simulink model "dc_motor_model_h_bridge_feedforward"  (Simulink 7.8)
settings: Solver=ode15s  StartTime=0.0  StopTime=10.0  MaxStep=1  RelTol=1e-3
values from neighbouring files (symbols this model uses):
  J = 8.85*10^(-7)    (= 8.85e-07)    [dc_motor_basic_blocks_feedforward.m]    (also in dc_motor_basic_blocks_feedforward_test.m; dc_motor_h_bridge_feedforward.m)
  T_load = 0.1    [dc_motor_basic_blocks_feedforward.m]    (also in dc_motor_basic_blocks_feedforward_test.m; dc_motor_h_bridge_feedforward.m)
  U_d = (R*mu/k_tau + k_emf) * w_d + R/k_tau * T_load + R*J/k_tau*w_d_dot    (= 34.1839823009)    [dc_motor_basic_blocks_feedforward.m]    (also in dc_motor_basic_blocks_feedforward_test.m; dc_motor_h_bridge_feedforward.m)
libraries: fl_lib x6, nesl_utility x6, elec_lib x3
settings Model: Creator=krzysztof  LastModifiedBy=krzysztof

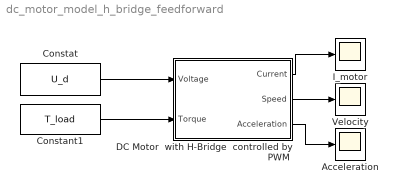
== system dc_motor_model_h_bridge_feedforward ==
  Acceleration : Scope
      settings: SaveName=Acceleration
  Constant1 : Constant  Value=T_load
  Constat : Constant  Value=U_d
  DC Motor  with H-Bridge  controlled by PWM : Subsystem
  I_motor : Scope
      settings: SaveName=i_motor
  Velocity : Scope
      settings: SaveName=w
  wires:
  DC Motor  with H-Bridge  controlled by PWM/1(Current) -> I_motor/1
  DC Motor  with H-Bridge  controlled by PWM/2(Speed) -> Velocity/1
  DC Motor  with H-Bridge  controlled by PWM/3(Acceleration) -> Acceleration/1
  Constat/1 -> DC Motor  with H-Bridge  controlled by PWM/1(Voltage)
  Constant1/1 -> DC Motor  with H-Bridge  controlled by PWM/2(Torque)

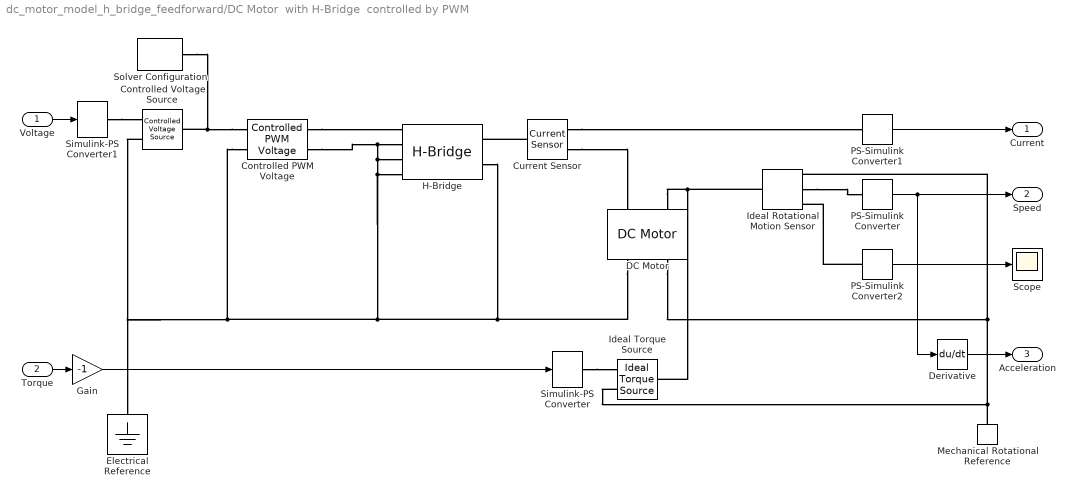
== system dc_motor_model_h_bridge_feedforward/DC Motor  with H-Bridge  controlled by PWM ==
  Voltage : Inport
  Torque : Inport  Port=2
  Controlled PWM Voltage : elec_lib/Actuators & Drivers/Drivers/Controlled PWM Voltage  F=f_PWM Hz  Vmin=Vmin V  Vmax=Vmax V  Vm=Vout V  pwm_or_av=2  current_Log=off  voltage_Log=off  power_Log=off  LocalVarNames=|current|voltage|power  LocalVarDescs=|Load current (A)|Load voltage (V)|Load power (W)  LocalVarLogging=[0 0 0]
  Controlled Voltage Source : fl_lib/Electrical/Electrical Sources/Controlled Voltage Source  i_Log=off  v_Log=off  LocalVarNames=|i|v  LocalVarDescs=|i|v  LocalVarLogging=[0 0]
  Current Sensor : fl_lib/Electrical/Electrical Sensors/Current Sensor  i1_Log=off  v1_Log=off  LocalVarNames=|i1|v1  LocalVarDescs=|i1|v1  LocalVarLogging=[0 0]
  DC Motor : elec_lib/Actuators & Drivers/Rotational Actuators/DC Motor  parameterization=2  Ra=3.9 Ohm  La=L H  emf_or_torque=1  Kv=7.2e-5 V/rpm  Ki=6.876e-4 N*m/A  T_stall=t_stall N*m  w_max=v_nl rad/s  w_rated=4070 rpm  P_rated=10 W  V_rated=Un V  J=J kg*m^2  lam_param=1  lam=mu N*m/(rad/s)  i_noload=I_nl A  V_i_noload=Un V  speed0=v0 rad/s  current_Log=off  voltage_Log=off  power_Log=off  i2r_Log=off  torque_Log=off  speed_Log=off  LocalVarNames=|current|voltage|power|i2r|torque|speed  LocalVarDescs=|Current (A)|Voltage (V)|Power (W)|Electrical losses (W)|Torque (Nm)|Angular speed (rad/s)  LocalVarLogging=[0 0 0 0 0 0]
  Derivative : Derivative
  Electrical Reference : fl_lib/Electrical/Electrical Elements/Electrical Reference  i_Log=off  LocalVarNames=|i  LocalVarDescs=|i  LocalVarLogging=0
  Gain : Gain  Gain=-1
  H-Bridge : elec_lib/Actuators & Drivers/Drivers/H-Bridge  Venable=in_en_tresh V  Vmax=in_pwm V  Vreverse=in_rev_tresh V  Vbrake=in_br_tresh V  Vm=h_Vout V  pwm_or_av=2  discontinuous=0  freewheeling_mode=1  freewheeling_mode_disc=1  Ron=h_res Ohm  Don=h_diode Ohm  Rload=10 Ohm  Lload=1e-5 H  F=10 kHz  current_Log=off  voltage_Log=off  power_Log=off  LocalVarNames=|current|voltage|power  LocalVarDescs=|Load current (A)|Load voltage (V)|Load power (W)  LocalVarLogging=[0 0 0]
  Ideal Rotational Motion Sensor : fl_lib/Mechanical/Mechanical Sensors/Ideal Rotational Motion Sensor  offset=0 rad  w_Log=off  t_Log=off  phi_Log=off  LocalVarNames=|w|t|phi  LocalVarDescs=|w|t|phi  LocalVarLogging=[0 0 0]
  Ideal Torque Source : fl_lib/Mechanical/Mechanical Sources/Ideal Torque Source  w_Log=off  t_Log=off  LocalVarNames=|w|t  LocalVarDescs=|w|t  LocalVarLogging=[0 0]
  Mechanical Rotational Reference : fl_lib/Mechanical/Rotational Elements/Mechanical Rotational Reference  t_Log=off  LocalVarNames=|t  LocalVarDescs=|t  LocalVarLogging=0
  PS-Simulink Converter : nesl_utility/PS-Simulink Converter  PhysicalDomain=network_engine_domain  LeftPortType=input  RightPortType=output  SubClassName=ps_output  Unit=rad/s  AffineConversion=off
  PS-Simulink Converter1 : nesl_utility/PS-Simulink Converter  PhysicalDomain=network_engine_domain  LeftPortType=input  RightPortType=output  SubClassName=ps_output  Unit=A  AffineConversion=off
  PS-Simulink Converter2 : nesl_utility/PS-Simulink Converter  PhysicalDomain=network_engine_domain  LeftPortType=input  RightPortType=output  SubClassName=ps_output  Unit=rad  AffineConversion=off
  Scope : Scope
  Simulink-PS Converter : nesl_utility/Simulink-PS Converter  PhysicalDomain=network_engine_domain  LeftPortType=input  RightPortType=output  SubClassName=ps_input  Unit=N*m  AffineConversion=off  InputFilterTimeConstant=.001  UdotUserProvided=0
  Simulink-PS Converter1 : nesl_utility/Simulink-PS Converter  PhysicalDomain=network_engine_domain  LeftPortType=input  RightPortType=output  SubClassName=ps_input  Unit=V  AffineConversion=off  InputFilterTimeConstant=.001  UdotUserProvided=0
  Solver Configuration : nesl_utility/Solver Configuration  PhysicalDomain=network_engine_domain  LeftPortType=input  RightPortType=generic  SubClassName=solver  DoDC=off  ResidualTolerance=1e-9  UseLocalSolver=off  LocalSolverChoice=NE_BACKWARD_EULER_ADVANCER  LocalSolverSampleTime=.001  DoFixedCost=off  MaxNonlinIter=3  MaxModeIter=2  LinearAlgebra=Sparse  Accelerate=off  Profile=off  UseLocalSampling=off  DelaysMemoryBudget=1024
  Current : Outport
  Speed : Outport  Port=2
  Acceleration : Outport  Port=3
  wires:
  Torque/1 -> Gain/1
  Voltage/1 -> Simulink-PS Converter1/1
  PS-Simulink Converter1/1 -> Current/1
  PS-Simulink Converter/1 -> Speed/1, Derivative/1
  PS-Simulink Converter2/1 -> Scope/1
  Derivative/1 -> Acceleration/1
  Gain/1 -> Simulink-PS Converter/1
  connections:
  Controlled PWM Voltage/LConn1 -- Solver Configuration/RConn1 -- Controlled Voltage Source/LConn1
  Controlled PWM Voltage/LConn2 -- DC Motor/RConn1 -- H-Bridge/RConn2 -- H-Bridge/LConn4 -- Controlled PWM Voltage/RConn2 -- H-Bridge/LConn2 -- H-Bridge/LConn3 -- Electrical Reference/LConn1 -- Controlled Voltage Source/RConn2
  Controlled PWM Voltage/RConn1 -- H-Bridge/LConn1
  Simulink-PS Converter1/RConn1 -- Controlled Voltage Source/RConn1
  Current Sensor/LConn1 -- H-Bridge/RConn1
  Current Sensor/RConn1 -- PS-Simulink Converter1/LConn1
  Current Sensor/RConn2 -- DC Motor/LConn1
  DC Motor/LConn2 -- Ideal Rotational Motion Sensor/LConn1 -- Ideal Torque Source/LConn1
  DC Motor/RConn2 -- Mechanical Rotational Reference/LConn1 -- Ideal Torque Source/RConn2 -- Ideal Rotational Motion Sensor/RConn1
  Ideal Rotational Motion Sensor/RConn2 -- PS-Simulink Converter/LConn1
  Simulink-PS Converter/RConn1 -- Ideal Torque Source/RConn1
  PS-Simulink Converter2/LConn1 -- Ideal Rotational Motion Sensor/RConn3
